simulink model "T3_updatesolarpart"  (R2022b)
settings: Solver=VariableStepAuto  StartTime=0.0  StopTime=10.0  RelTol=1e-3
undefined symbols (not defined in the file): High, Low
libraries: fl_lib x101, nesl_utility x52, simulink x14, ee_lib x5, slpidlib x2, eePwmGenerator x1
(part 2 of 3)

== system T3_updatesolarpart/Household 9 ==
  Current Sensor : fl_lib/Electrical/Electrical Sensors/Current Sensor
  PS-Simulink Converter : nesl_utility/PS-Simulink Converter  PhysicalDomain=network_engine_domain  SubClassName=ps_output  LeftPortType=input  RightPortType=output  PseudoPeriodic=off  Frequencies=[]  VectorFormat=inherit  Unit=inherit  AffineConversion=off
  PS-Simulink Converter1 : nesl_utility/PS-Simulink Converter  PhysicalDomain=network_engine_domain  SubClassName=ps_output  LeftPortType=input  RightPortType=output  PseudoPeriodic=off  Frequencies=[]  VectorFormat=inherit  Unit=inherit  AffineConversion=off
  Product : Product
  "Residential power " : simulink/Sources/Repeating Sequence Interpolated  OutValues=[2.8 2.5 2 2 2.2 2.5 2.8 3.4 3.6 3.8 4 4 4 4 4 4 4 4 4 4 3.8 3.5 3.2 3]*1000  TimeValues=[0 1 2 3 4 5 6 7 8 9 10 11 12 13 14 15 16 17 18 19 20 21 22 23]  LookUpMeth=Interpolation-Use End Values  tsamp=1e-4  OutMin=[]  OutMax=[]  OutDataTypeStr=double  OutputDataTypeScalingMode=double  OutDataType=fixdt(0,8)  OutScaling=2^-10
  Simscape Component : SimscapeComponentBlock  SourceFile=ResidentialPowerLoad  ComponentPath=ResidentialPowerLoad  ComponentVariants="[\"ResidentialPowerLoad\"]"  ComponentVariantNames="[\"ResidentialPowerLoad\"]"  ClassName=ResidentialPowerLoad  SchemaVersion=1  i_specify=off  i_priority=None  i=0 A  i_nominal_specify=off  i_nominal_unit=A  i_nominal_value=1  v_specify=off  v_priority=None  v=0 V  v_nominal_specify=off  v_nominal_unit=V  v_nominal_value=1
      settings: CopyFcn=simscape.engine.sli.internal.componentblockcallback(gcbh,'COPY')  PreCopyFcn=simscape.engine.sli.internal.componentblockcallback(gcbh,'PRECOPY')  PreDeleteFcn=simscape.engine.sli.internal.componentblockcallback(gcbh,'PREDELETE')  InternalSimscapePortConfiguration="{\"Bottom\":[],\"Left\":[{\"id\":\"Power\",\"label\":\"P\",\"type\":\"input\"},{\"id\":\"p\",\"label\":\"+\",\"type\":\"foundation.electrical.electrical\"}],\"Right\":[{\"id\":\"n\",\"label\":\"-\",\"type\":\"foundation.electrical.electrical\"}],\"Top\":[]}"
      mask Type: ResidentialPowerLoad
      mask Display: color('red');plot([0 1 1 0 0],[0 0 1 1 0]);plot([0.7,1],[1,0.7]);plot(-2,-1.75);plot(3, 1);disp('\n.ssc\nUnresolved')
  Simscape Bus1 : SimscapeBus  HierarchyStrings=High;Low
  Simulink-PS Converter : nesl_utility/Simulink-PS Converter  PhysicalDomain=network_engine_domain  SubClassName=ps_input  LeftPortType=input  RightPortType=output  PseudoPeriodic=off  Frequencies=[]  NoiseDistribution=none  NoiseParameters=[]  Unit=1  AffineConversion=off  FilteringAndDerivatives=provide  SimscapeFilterOrder=1  InputFilterTimeConstant=0.001  UdotUserProvided=0
  Terminator : Terminator
  Voltage Sensor : fl_lib/Electrical/Electrical Sensors/Voltage Sensor
  ResidentialOut : PMIOPort  Side=Right
  wires:
  Product/1 -> Terminator/1  "power"
  PS-Simulink Converter1/1 -> Product/1  "current"
  PS-Simulink Converter/1 -> Product/2  "voltage"
  "Residential power "/1 -> Simulink-PS Converter/1
  connections:
  Current Sensor/RConn1 -- PS-Simulink Converter1/LConn1
  Current Sensor/LConn1 -- Simscape Bus1/LConn1
  Simulink-PS Converter/RConn1 -- Simscape Component/LConn1
  Voltage Sensor/RConn1 -- PS-Simulink Converter/LConn1
  Voltage Sensor/LConn1 -- Current Sensor/RConn2 -- Simscape Component/LConn2
  ResidentialOut/RConn1 -- Simscape Bus1/RConn1
  Simscape Component/RConn1 -- Simscape Bus1/LConn2 -- Voltage Sensor/RConn2

== system T3_updatesolarpart/Line1 ==
  Resistor : fl_lib/Electrical/Electrical Elements/Resistor  R=rho*l/A Ohm  i_specify=off  i_priority=None  i=0 A  i_nominal_specify=off  i_nominal_unit=A  i_nominal_value=1  v_specify=off  v_priority=None  v=0 V  v_nominal_specify=off  v_nominal_unit=V  v_nominal_value=1
  Resistor1 : fl_lib/Electrical/Electrical Elements/Resistor  R=rho*l/A Ohm  i_specify=off  i_priority=None  i=0 A  i_nominal_specify=off  i_nominal_unit=A  i_nominal_value=1  v_specify=off  v_priority=None  v=0 V  v_nominal_specify=off  v_nominal_unit=V  v_nominal_value=1
  Simscape Bus2 : SimscapeBus  HierarchyStrings=High;Low
  Simscape Bus3 : SimscapeBus  HierarchyStrings=High;Low
  In : PMIOPort  Side=Left
  Out : PMIOPort  Port=2  Side=Right
  connections:
  Simscape Bus2/LConn1 -- Resistor/LConn1
  Simscape Bus3/LConn2 -- Resistor1/RConn1
  Simscape Bus2/RConn1 -- In/RConn1
  Simscape Bus3/LConn1 -- Resistor/RConn1
  Resistor1/LConn1 -- Simscape Bus2/LConn2
  Simscape Bus3/RConn1 -- Out/RConn1

== system T3_updatesolarpart/Line10 ==
  Resistor : fl_lib/Electrical/Electrical Elements/Resistor  R=rho*l/A Ohm  i_specify=off  i_priority=None  i=0 A  i_nominal_specify=off  i_nominal_unit=A  i_nominal_value=1  v_specify=off  v_priority=None  v=0 V  v_nominal_specify=off  v_nominal_unit=V  v_nominal_value=1
  Resistor1 : fl_lib/Electrical/Electrical Elements/Resistor  R=rho*l/A Ohm  i_specify=off  i_priority=None  i=0 A  i_nominal_specify=off  i_nominal_unit=A  i_nominal_value=1  v_specify=off  v_priority=None  v=0 V  v_nominal_specify=off  v_nominal_unit=V  v_nominal_value=1
  Simscape Bus2 : SimscapeBus  HierarchyStrings=High;Low
  Simscape Bus3 : SimscapeBus  HierarchyStrings=High;Low
  In : PMIOPort  Side=Left
  Out : PMIOPort  Port=2  Side=Right
  connections:
  Simscape Bus2/LConn1 -- Resistor/LConn1
  Simscape Bus3/LConn2 -- Resistor1/RConn1
  Simscape Bus2/RConn1 -- In/RConn1
  Simscape Bus3/LConn1 -- Resistor/RConn1
  Resistor1/LConn1 -- Simscape Bus2/LConn2
  Simscape Bus3/RConn1 -- Out/RConn1

== system T3_updatesolarpart/Line11 ==
  Resistor : fl_lib/Electrical/Electrical Elements/Resistor  R=rho*l/A Ohm  i_specify=off  i_priority=None  i=0 A  i_nominal_specify=off  i_nominal_unit=A  i_nominal_value=1  v_specify=off  v_priority=None  v=0 V  v_nominal_specify=off  v_nominal_unit=V  v_nominal_value=1
  Resistor1 : fl_lib/Electrical/Electrical Elements/Resistor  R=rho*l/A Ohm  i_specify=off  i_priority=None  i=0 A  i_nominal_specify=off  i_nominal_unit=A  i_nominal_value=1  v_specify=off  v_priority=None  v=0 V  v_nominal_specify=off  v_nominal_unit=V  v_nominal_value=1
  Simscape Bus2 : SimscapeBus  HierarchyStrings=High;Low
  Simscape Bus3 : SimscapeBus  HierarchyStrings=High;Low
  In : PMIOPort  Side=Left
  Out : PMIOPort  Port=2  Side=Right
  connections:
  Simscape Bus3/RConn1 -- Out/RConn1
  Resistor1/LConn1 -- Simscape Bus2/LConn2
  Simscape Bus3/LConn1 -- Resistor/RConn1
  Simscape Bus2/RConn1 -- In/RConn1
  Simscape Bus3/LConn2 -- Resistor1/RConn1
  Simscape Bus2/LConn1 -- Resistor/LConn1

== system T3_updatesolarpart/Line12 ==
  Resistor : fl_lib/Electrical/Electrical Elements/Resistor  R=rho*l/A Ohm  i_specify=off  i_priority=None  i=0 A  i_nominal_specify=off  i_nominal_unit=A  i_nominal_value=1  v_specify=off  v_priority=None  v=0 V  v_nominal_specify=off  v_nominal_unit=V  v_nominal_value=1
  Resistor1 : fl_lib/Electrical/Electrical Elements/Resistor  R=rho*l/A Ohm  i_specify=off  i_priority=None  i=0 A  i_nominal_specify=off  i_nominal_unit=A  i_nominal_value=1  v_specify=off  v_priority=None  v=0 V  v_nominal_specify=off  v_nominal_unit=V  v_nominal_value=1
  Simscape Bus2 : SimscapeBus  HierarchyStrings=High;Low
  Simscape Bus3 : SimscapeBus  HierarchyStrings=High;Low
  In : PMIOPort  Side=Left
  Out : PMIOPort  Port=2  Side=Right
  connections:
  Simscape Bus3/RConn1 -- Out/RConn1
  Resistor1/LConn1 -- Simscape Bus2/LConn2
  Simscape Bus3/LConn1 -- Resistor/RConn1
  Simscape Bus2/RConn1 -- In/RConn1
  Simscape Bus3/LConn2 -- Resistor1/RConn1
  Simscape Bus2/LConn1 -- Resistor/LConn1

== system T3_updatesolarpart/Line13 ==
  Resistor : fl_lib/Electrical/Electrical Elements/Resistor  R=rho*l/A Ohm  i_specify=off  i_priority=None  i=0 A  i_nominal_specify=off  i_nominal_unit=A  i_nominal_value=1  v_specify=off  v_priority=None  v=0 V  v_nominal_specify=off  v_nominal_unit=V  v_nominal_value=1
  Resistor1 : fl_lib/Electrical/Electrical Elements/Resistor  R=rho*l/A Ohm  i_specify=off  i_priority=None  i=0 A  i_nominal_specify=off  i_nominal_unit=A  i_nominal_value=1  v_specify=off  v_priority=None  v=0 V  v_nominal_specify=off  v_nominal_unit=V  v_nominal_value=1
  Simscape Bus2 : SimscapeBus  HierarchyStrings=High;Low
  Simscape Bus3 : SimscapeBus  HierarchyStrings=High;Low
  In : PMIOPort  Side=Left
  Out : PMIOPort  Port=2  Side=Right
  connections:
  Simscape Bus2/LConn1 -- Resistor/LConn1
  Simscape Bus3/LConn2 -- Resistor1/RConn1
  Simscape Bus2/RConn1 -- In/RConn1
  Simscape Bus3/LConn1 -- Resistor/RConn1
  Resistor1/LConn1 -- Simscape Bus2/LConn2
  Simscape Bus3/RConn1 -- Out/RConn1

== system T3_updatesolarpart/Line14 ==
  Resistor : fl_lib/Electrical/Electrical Elements/Resistor  R=rho*l/A Ohm  i_specify=off  i_priority=None  i=0 A  i_nominal_specify=off  i_nominal_unit=A  i_nominal_value=1  v_specify=off  v_priority=None  v=0 V  v_nominal_specify=off  v_nominal_unit=V  v_nominal_value=1
  Resistor1 : fl_lib/Electrical/Electrical Elements/Resistor  R=rho*l/A Ohm  i_specify=off  i_priority=None  i=0 A  i_nominal_specify=off  i_nominal_unit=A  i_nominal_value=1  v_specify=off  v_priority=None  v=0 V  v_nominal_specify=off  v_nominal_unit=V  v_nominal_value=1
  Simscape Bus2 : SimscapeBus  HierarchyStrings=High;Low
  Simscape Bus3 : SimscapeBus  HierarchyStrings=High;Low
  In : PMIOPort  Side=Left
  Out : PMIOPort  Port=2  Side=Right
  connections:
  Simscape Bus3/RConn1 -- Out/RConn1
  Resistor1/LConn1 -- Simscape Bus2/LConn2
  Simscape Bus3/LConn1 -- Resistor/RConn1
  Simscape Bus2/RConn1 -- In/RConn1
  Simscape Bus3/LConn2 -- Resistor1/RConn1
  Simscape Bus2/LConn1 -- Resistor/LConn1

== system T3_updatesolarpart/Line15 ==
  Resistor : fl_lib/Electrical/Electrical Elements/Resistor  R=rho*l/A Ohm  i_specify=off  i_priority=None  i=0 A  i_nominal_specify=off  i_nominal_unit=A  i_nominal_value=1  v_specify=off  v_priority=None  v=0 V  v_nominal_specify=off  v_nominal_unit=V  v_nominal_value=1
  Resistor1 : fl_lib/Electrical/Electrical Elements/Resistor  R=rho*l/A Ohm  i_specify=off  i_priority=None  i=0 A  i_nominal_specify=off  i_nominal_unit=A  i_nominal_value=1  v_specify=off  v_priority=None  v=0 V  v_nominal_specify=off  v_nominal_unit=V  v_nominal_value=1
  Simscape Bus2 : SimscapeBus  HierarchyStrings=High;Low
  Simscape Bus3 : SimscapeBus  HierarchyStrings=High;Low
  In : PMIOPort  Side=Left
  Out : PMIOPort  Port=2  Side=Right
  connections:
  Simscape Bus2/LConn1 -- Resistor/LConn1
  Simscape Bus3/LConn2 -- Resistor1/RConn1
  Simscape Bus2/RConn1 -- In/RConn1
  Simscape Bus3/LConn1 -- Resistor/RConn1
  Resistor1/LConn1 -- Simscape Bus2/LConn2
  Simscape Bus3/RConn1 -- Out/RConn1

== system T3_updatesolarpart/Line16 ==
  Resistor : fl_lib/Electrical/Electrical Elements/Resistor  R=rho*l/A Ohm  i_specify=off  i_priority=None  i=0 A  i_nominal_specify=off  i_nominal_unit=A  i_nominal_value=1  v_specify=off  v_priority=None  v=0 V  v_nominal_specify=off  v_nominal_unit=V  v_nominal_value=1
  Resistor1 : fl_lib/Electrical/Electrical Elements/Resistor  R=rho*l/A Ohm  i_specify=off  i_priority=None  i=0 A  i_nominal_specify=off  i_nominal_unit=A  i_nominal_value=1  v_specify=off  v_priority=None  v=0 V  v_nominal_specify=off  v_nominal_unit=V  v_nominal_value=1
  Simscape Bus2 : SimscapeBus  HierarchyStrings=High;Low
  Simscape Bus3 : SimscapeBus  HierarchyStrings=High;Low
  In : PMIOPort  Side=Left
  Out : PMIOPort  Port=2  Side=Right
  connections:
  Simscape Bus2/LConn1 -- Resistor/LConn1
  Simscape Bus3/LConn2 -- Resistor1/RConn1
  Simscape Bus2/RConn1 -- In/RConn1
  Simscape Bus3/LConn1 -- Resistor/RConn1
  Resistor1/LConn1 -- Simscape Bus2/LConn2
  Simscape Bus3/RConn1 -- Out/RConn1

== system T3_updatesolarpart/Line17 ==
  Resistor : fl_lib/Electrical/Electrical Elements/Resistor  R=rho*l/A Ohm  i_specify=off  i_priority=None  i=0 A  i_nominal_specify=off  i_nominal_unit=A  i_nominal_value=1  v_specify=off  v_priority=None  v=0 V  v_nominal_specify=off  v_nominal_unit=V  v_nominal_value=1
  Resistor1 : fl_lib/Electrical/Electrical Elements/Resistor  R=rho*l/A Ohm  i_specify=off  i_priority=None  i=0 A  i_nominal_specify=off  i_nominal_unit=A  i_nominal_value=1  v_specify=off  v_priority=None  v=0 V  v_nominal_specify=off  v_nominal_unit=V  v_nominal_value=1
  Simscape Bus2 : SimscapeBus  HierarchyStrings=High;Low
  Simscape Bus3 : SimscapeBus  HierarchyStrings=High;Low
  In : PMIOPort  Side=Left
  Out : PMIOPort  Port=2  Side=Right
  connections:
  Simscape Bus3/RConn1 -- Out/RConn1
  Resistor1/LConn1 -- Simscape Bus2/LConn2
  Simscape Bus3/LConn1 -- Resistor/RConn1
  Simscape Bus2/RConn1 -- In/RConn1
  Simscape Bus3/LConn2 -- Resistor1/RConn1
  Simscape Bus2/LConn1 -- Resistor/LConn1

== system T3_updatesolarpart/Line18 ==
  Resistor : fl_lib/Electrical/Electrical Elements/Resistor  R=rho*l/A Ohm  i_specify=off  i_priority=None  i=0 A  i_nominal_specify=off  i_nominal_unit=A  i_nominal_value=1  v_specify=off  v_priority=None  v=0 V  v_nominal_specify=off  v_nominal_unit=V  v_nominal_value=1
  Resistor1 : fl_lib/Electrical/Electrical Elements/Resistor  R=rho*l/A Ohm  i_specify=off  i_priority=None  i=0 A  i_nominal_specify=off  i_nominal_unit=A  i_nominal_value=1  v_specify=off  v_priority=None  v=0 V  v_nominal_specify=off  v_nominal_unit=V  v_nominal_value=1
  Simscape Bus2 : SimscapeBus  HierarchyStrings=High;Low
  Simscape Bus3 : SimscapeBus  HierarchyStrings=High;Low
  In : PMIOPort  Side=Left
  Out : PMIOPort  Port=2  Side=Right
  connections:
  Simscape Bus3/RConn1 -- Out/RConn1
  Resistor1/LConn1 -- Simscape Bus2/LConn2
  Simscape Bus3/LConn1 -- Resistor/RConn1
  Simscape Bus2/RConn1 -- In/RConn1
  Simscape Bus3/LConn2 -- Resistor1/RConn1
  Simscape Bus2/LConn1 -- Resistor/LConn1

== system T3_updatesolarpart/Line19 ==
  Resistor : fl_lib/Electrical/Electrical Elements/Resistor  R=rho*l/A Ohm  i_specify=off  i_priority=None  i=0 A  i_nominal_specify=off  i_nominal_unit=A  i_nominal_value=1  v_specify=off  v_priority=None  v=0 V  v_nominal_specify=off  v_nominal_unit=V  v_nominal_value=1
  Resistor1 : fl_lib/Electrical/Electrical Elements/Resistor  R=rho*l/A Ohm  i_specify=off  i_priority=None  i=0 A  i_nominal_specify=off  i_nominal_unit=A  i_nominal_value=1  v_specify=off  v_priority=None  v=0 V  v_nominal_specify=off  v_nominal_unit=V  v_nominal_value=1
  Simscape Bus2 : SimscapeBus  HierarchyStrings=High;Low
  Simscape Bus3 : SimscapeBus  HierarchyStrings=High;Low
  In : PMIOPort  Side=Left
  Out : PMIOPort  Port=2  Side=Right
  connections:
  Simscape Bus2/LConn1 -- Resistor/LConn1
  Simscape Bus3/LConn2 -- Resistor1/RConn1
  Simscape Bus2/RConn1 -- In/RConn1
  Simscape Bus3/LConn1 -- Resistor/RConn1
  Resistor1/LConn1 -- Simscape Bus2/LConn2
  Simscape Bus3/RConn1 -- Out/RConn1

== system T3_updatesolarpart/Line2 ==
  Resistor : fl_lib/Electrical/Electrical Elements/Resistor  R=rho*l/A Ohm  i_specify=off  i_priority=None  i=0 A  i_nominal_specify=off  i_nominal_unit=A  i_nominal_value=1  v_specify=off  v_priority=None  v=0 V  v_nominal_specify=off  v_nominal_unit=V  v_nominal_value=1
  Resistor1 : fl_lib/Electrical/Electrical Elements/Resistor  R=rho*l/A Ohm  i_specify=off  i_priority=None  i=0 A  i_nominal_specify=off  i_nominal_unit=A  i_nominal_value=1  v_specify=off  v_priority=None  v=0 V  v_nominal_specify=off  v_nominal_unit=V  v_nominal_value=1
  Simscape Bus2 : SimscapeBus  HierarchyStrings=High;Low
  Simscape Bus3 : SimscapeBus  HierarchyStrings=High;Low
  In : PMIOPort  Side=Left
  Out : PMIOPort  Port=2  Side=Right
  connections:
  Simscape Bus3/RConn1 -- Out/RConn1
  Resistor1/LConn1 -- Simscape Bus2/LConn2
  Simscape Bus3/LConn1 -- Resistor/RConn1
  Simscape Bus2/RConn1 -- In/RConn1
  Simscape Bus3/LConn2 -- Resistor1/RConn1
  Simscape Bus2/LConn1 -- Resistor/LConn1

== system T3_updatesolarpart/Line20 ==
  Resistor : fl_lib/Electrical/Electrical Elements/Resistor  R=rho*l/A Ohm  i_specify=off  i_priority=None  i=0 A  i_nominal_specify=off  i_nominal_unit=A  i_nominal_value=1  v_specify=off  v_priority=None  v=0 V  v_nominal_specify=off  v_nominal_unit=V  v_nominal_value=1
  Resistor1 : fl_lib/Electrical/Electrical Elements/Resistor  R=rho*l/A Ohm  i_specify=off  i_priority=None  i=0 A  i_nominal_specify=off  i_nominal_unit=A  i_nominal_value=1  v_specify=off  v_priority=None  v=0 V  v_nominal_specify=off  v_nominal_unit=V  v_nominal_value=1
  Simscape Bus2 : SimscapeBus  HierarchyStrings=High;Low
  Simscape Bus3 : SimscapeBus  HierarchyStrings=High;Low
  In : PMIOPort  Side=Left
  Out : PMIOPort  Port=2  Side=Right
  connections:
  Simscape Bus3/RConn1 -- Out/RConn1
  Resistor1/LConn1 -- Simscape Bus2/LConn2
  Simscape Bus3/LConn1 -- Resistor/RConn1
  Simscape Bus2/RConn1 -- In/RConn1
  Simscape Bus3/LConn2 -- Resistor1/RConn1
  Simscape Bus2/LConn1 -- Resistor/LConn1

== system T3_updatesolarpart/Line3 ==
  Resistor : fl_lib/Electrical/Electrical Elements/Resistor  R=rho*l/A Ohm  i_specify=off  i_priority=None  i=0 A  i_nominal_specify=off  i_nominal_unit=A  i_nominal_value=1  v_specify=off  v_priority=None  v=0 V  v_nominal_specify=off  v_nominal_unit=V  v_nominal_value=1
  Resistor1 : fl_lib/Electrical/Electrical Elements/Resistor  R=rho*l/A Ohm  i_specify=off  i_priority=None  i=0 A  i_nominal_specify=off  i_nominal_unit=A  i_nominal_value=1  v_specify=off  v_priority=None  v=0 V  v_nominal_specify=off  v_nominal_unit=V  v_nominal_value=1
  Simscape Bus2 : SimscapeBus  HierarchyStrings=High;Low
  Simscape Bus3 : SimscapeBus  HierarchyStrings=High;Low
  In : PMIOPort  Side=Left
  Out : PMIOPort  Port=2  Side=Right
  connections:
  Simscape Bus2/LConn1 -- Resistor/LConn1
  Simscape Bus3/LConn2 -- Resistor1/RConn1
  Simscape Bus2/RConn1 -- In/RConn1
  Simscape Bus3/LConn1 -- Resistor/RConn1
  Resistor1/LConn1 -- Simscape Bus2/LConn2
  Simscape Bus3/RConn1 -- Out/RConn1

== system T3_updatesolarpart/Line4 ==
  Resistor : fl_lib/Electrical/Electrical Elements/Resistor  R=rho*l/A Ohm  i_specify=off  i_priority=None  i=0 A  i_nominal_specify=off  i_nominal_unit=A  i_nominal_value=1  v_specify=off  v_priority=None  v=0 V  v_nominal_specify=off  v_nominal_unit=V  v_nominal_value=1
  Resistor1 : fl_lib/Electrical/Electrical Elements/Resistor  R=rho*l/A Ohm  i_specify=off  i_priority=None  i=0 A  i_nominal_specify=off  i_nominal_unit=A  i_nominal_value=1  v_specify=off  v_priority=None  v=0 V  v_nominal_specify=off  v_nominal_unit=V  v_nominal_value=1
  Simscape Bus2 : SimscapeBus  HierarchyStrings=High;Low
  Simscape Bus3 : SimscapeBus  HierarchyStrings=High;Low
  In : PMIOPort  Side=Left
  Out : PMIOPort  Port=2  Side=Right
  connections:
  Simscape Bus3/RConn1 -- Out/RConn1
  Resistor1/LConn1 -- Simscape Bus2/LConn2
  Simscape Bus3/LConn1 -- Resistor/RConn1
  Simscape Bus2/RConn1 -- In/RConn1
  Simscape Bus3/LConn2 -- Resistor1/RConn1
  Simscape Bus2/LConn1 -- Resistor/LConn1

== system T3_updatesolarpart/Line5 ==
  Resistor : fl_lib/Electrical/Electrical Elements/Resistor  R=rho*l/A Ohm  i_specify=off  i_priority=None  i=0 A  i_nominal_specify=off  i_nominal_unit=A  i_nominal_value=1  v_specify=off  v_priority=None  v=0 V  v_nominal_specify=off  v_nominal_unit=V  v_nominal_value=1
  Resistor1 : fl_lib/Electrical/Electrical Elements/Resistor  R=rho*l/A Ohm  i_specify=off  i_priority=None  i=0 A  i_nominal_specify=off  i_nominal_unit=A  i_nominal_value=1  v_specify=off  v_priority=None  v=0 V  v_nominal_specify=off  v_nominal_unit=V  v_nominal_value=1
  Simscape Bus2 : SimscapeBus  HierarchyStrings=High;Low
  Simscape Bus3 : SimscapeBus  HierarchyStrings=High;Low
  In : PMIOPort  Side=Left
  Out : PMIOPort  Port=2  Side=Right
  connections:
  Simscape Bus2/LConn1 -- Resistor/LConn1
  Simscape Bus3/LConn2 -- Resistor1/RConn1
  Simscape Bus2/RConn1 -- In/RConn1
  Simscape Bus3/LConn1 -- Resistor/RConn1
  Resistor1/LConn1 -- Simscape Bus2/LConn2
  Simscape Bus3/RConn1 -- Out/RConn1

== system T3_updatesolarpart/Line6 ==
  Resistor : fl_lib/Electrical/Electrical Elements/Resistor  R=rho*l/A Ohm  i_specify=off  i_priority=None  i=0 A  i_nominal_specify=off  i_nominal_unit=A  i_nominal_value=1  v_specify=off  v_priority=None  v=0 V  v_nominal_specify=off  v_nominal_unit=V  v_nominal_value=1
  Resistor1 : fl_lib/Electrical/Electrical Elements/Resistor  R=rho*l/A Ohm  i_specify=off  i_priority=None  i=0 A  i_nominal_specify=off  i_nominal_unit=A  i_nominal_value=1  v_specify=off  v_priority=None  v=0 V  v_nominal_specify=off  v_nominal_unit=V  v_nominal_value=1
  Simscape Bus2 : SimscapeBus  HierarchyStrings=High;Low
  Simscape Bus3 : SimscapeBus  HierarchyStrings=High;Low
  In : PMIOPort  Side=Left
  Out : PMIOPort  Port=2  Side=Right
  connections:
  Simscape Bus3/RConn1 -- Out/RConn1
  Resistor1/LConn1 -- Simscape Bus2/LConn2
  Simscape Bus3/LConn1 -- Resistor/RConn1
  Simscape Bus2/RConn1 -- In/RConn1
  Simscape Bus3/LConn2 -- Resistor1/RConn1
  Simscape Bus2/LConn1 -- Resistor/LConn1

== system T3_updatesolarpart/Line7 ==
  Resistor : fl_lib/Electrical/Electrical Elements/Resistor  R=rho*l/A Ohm  i_specify=off  i_priority=None  i=0 A  i_nominal_specify=off  i_nominal_unit=A  i_nominal_value=1  v_specify=off  v_priority=None  v=0 V  v_nominal_specify=off  v_nominal_unit=V  v_nominal_value=1
  Resistor1 : fl_lib/Electrical/Electrical Elements/Resistor  R=rho*l/A Ohm  i_specify=off  i_priority=None  i=0 A  i_nominal_specify=off  i_nominal_unit=A  i_nominal_value=1  v_specify=off  v_priority=None  v=0 V  v_nominal_specify=off  v_nominal_unit=V  v_nominal_value=1
  Simscape Bus2 : SimscapeBus  HierarchyStrings=High;Low
  Simscape Bus3 : SimscapeBus  HierarchyStrings=High;Low
  In : PMIOPort  Side=Left
  Out : PMIOPort  Port=2  Side=Right
  connections:
  Simscape Bus2/LConn1 -- Resistor/LConn1
  Simscape Bus3/LConn2 -- Resistor1/RConn1
  Simscape Bus2/RConn1 -- In/RConn1
  Simscape Bus3/LConn1 -- Resistor/RConn1
  Resistor1/LConn1 -- Simscape Bus2/LConn2
  Simscape Bus3/RConn1 -- Out/RConn1

== system T3_updatesolarpart/Line8 ==
  Resistor : fl_lib/Electrical/Electrical Elements/Resistor  R=rho*l/A Ohm  i_specify=off  i_priority=None  i=0 A  i_nominal_specify=off  i_nominal_unit=A  i_nominal_value=1  v_specify=off  v_priority=None  v=0 V  v_nominal_specify=off  v_nominal_unit=V  v_nominal_value=1
  Resistor1 : fl_lib/Electrical/Electrical Elements/Resistor  R=rho*l/A Ohm  i_specify=off  i_priority=None  i=0 A  i_nominal_specify=off  i_nominal_unit=A  i_nominal_value=1  v_specify=off  v_priority=None  v=0 V  v_nominal_specify=off  v_nominal_unit=V  v_nominal_value=1
  Simscape Bus2 : SimscapeBus  HierarchyStrings=High;Low
  Simscape Bus3 : SimscapeBus  HierarchyStrings=High;Low
  In : PMIOPort  Side=Left
  Out : PMIOPort  Port=2  Side=Right
  connections:
  Simscape Bus2/LConn1 -- Resistor/LConn1
  Simscape Bus3/LConn2 -- Resistor1/RConn1
  Simscape Bus2/RConn1 -- In/RConn1
  Simscape Bus3/LConn1 -- Resistor/RConn1
  Resistor1/LConn1 -- Simscape Bus2/LConn2
  Simscape Bus3/RConn1 -- Out/RConn1

== system T3_updatesolarpart/Line9 ==
  Resistor : fl_lib/Electrical/Electrical Elements/Resistor  R=rho*l/A Ohm  i_specify=off  i_priority=None  i=0 A  i_nominal_specify=off  i_nominal_unit=A  i_nominal_value=1  v_specify=off  v_priority=None  v=0 V  v_nominal_specify=off  v_nominal_unit=V  v_nominal_value=1
  Resistor1 : fl_lib/Electrical/Electrical Elements/Resistor  R=rho*l/A Ohm  i_specify=off  i_priority=None  i=0 A  i_nominal_specify=off  i_nominal_unit=A  i_nominal_value=1  v_specify=off  v_priority=None  v=0 V  v_nominal_specify=off  v_nominal_unit=V  v_nominal_value=1
  Simscape Bus2 : SimscapeBus  HierarchyStrings=High;Low
  Simscape Bus3 : SimscapeBus  HierarchyStrings=High;Low
  In : PMIOPort  Side=Left
  Out : PMIOPort  Port=2  Side=Right
  connections:
  Simscape Bus3/RConn1 -- Out/RConn1
  Resistor1/LConn1 -- Simscape Bus2/LConn2
  Simscape Bus3/LConn1 -- Resistor/RConn1
  Simscape Bus2/RConn1 -- In/RConn1
  Simscape Bus3/LConn2 -- Resistor1/RConn1
  Simscape Bus2/LConn1 -- Resistor/LConn1

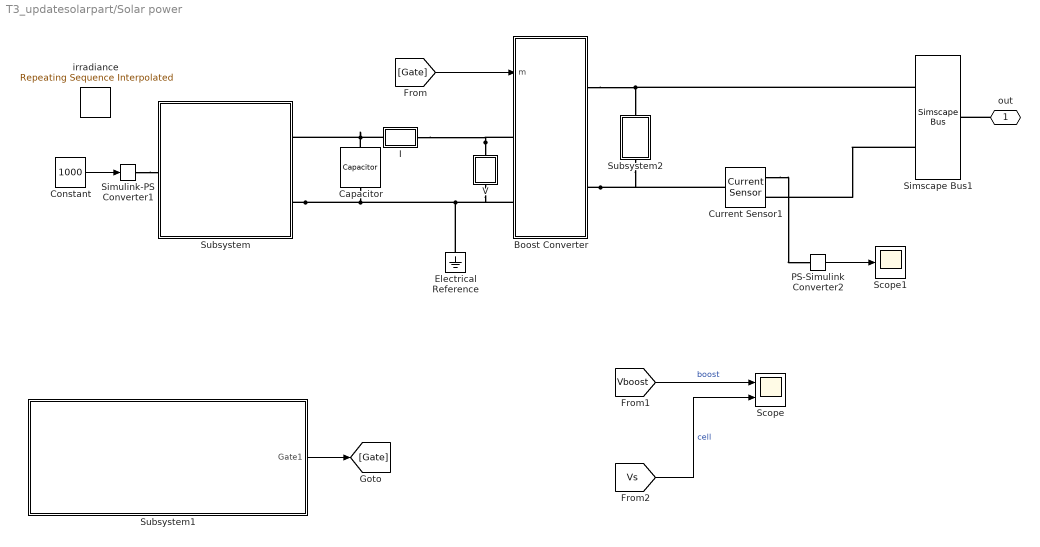
== system T3_updatesolarpart/Solar power ==
  Boost Converter : Subsystem  VariantControl=boostCircuit == 1
  Capacitor : fl_lib/Electrical/Electrical Elements/Capacitor  c=1e-3 F  r=1e-6 Ohm  g=0 1/Ohm  i_specify=off  i_priority=None  i=0 A  i_nominal_specify=off  i_nominal_unit=A  i_nominal_value=1  v_specify=off  v_priority=None  v=0 V  v_nominal_specify=off  v_nominal_unit=V  v_nominal_value=1  vc_specify=off  vc_priority=High  vc=0 V  vc_nominal_specify=off  vc_nominal_unit=V  vc_nominal_value=1
  Constant : Constant  Value=1000  SampleTime=20e3
  Current Sensor1 : fl_lib/Electrical/Electrical Sensors/Current Sensor
  Electrical Reference : fl_lib/Electrical/Electrical Elements/Electrical Reference
  I : Subsystem
  PS-Simulink Converter2 : nesl_utility/PS-Simulink Converter  PhysicalDomain=network_engine_domain  SubClassName=ps_output  LeftPortType=input  RightPortType=output  PseudoPeriodic=off  Frequencies=[]  VectorFormat=inherit  Unit=inherit  AffineConversion=off
  Scope : Scope  NumInputPorts=2
  Scope1 : Scope
  Simscape Bus1 : SimscapeBus  HierarchyStrings=High;Low
  Simulink-PS Converter1 : nesl_utility/Simulink-PS Converter  PhysicalDomain=network_engine_domain  SubClassName=ps_input  LeftPortType=input  RightPortType=output  PseudoPeriodic=off  Frequencies=[]  NoiseDistribution=none  NoiseParameters=[]  Unit=1  AffineConversion=off  FilteringAndDerivatives=provide  SimscapeFilterOrder=1  InputFilterTimeConstant=0.001  UdotUserProvided=0
  Subsystem : Subsystem
  Subsystem1 : Subsystem
  Subsystem2 : Subsystem
  V : Subsystem
  "irradiance " : simulink/Sources/Repeating Sequence Interpolated  OutValues=[0 0 1 1 2 2 3 3 4 4 5 5 6 6 5 5 4 4 3 3 2 2 1 1]*200  TimeValues=[0 1 2 3 4 5 6 7 8 9 10 11 12 13 14 15 16 17 18 19 20 21 22 23]  LookUpMeth=Interpolation-Use End Values  tsamp=1e-4  OutMin=[]  OutMax=[]  OutDataTypeStr=double  OutputDataTypeScalingMode=double  OutDataType=fixdt(0,8)  OutScaling=2^-10
  out : PMIOPort  Side=Left
  wires:
  [Vs] -> Scope/2  "cell"
  [Gate] -> Boost Converter/1(m)
  [Vboost] -> Scope/1  "boost"
  Constant/1 -> Simulink-PS Converter1/1
  Subsystem1/1(Gate1) -> [Gate]
  PS-Simulink Converter2/1 -> Scope1/1
  connections:
  out/RConn1 -- Simscape Bus1/RConn1
  Subsystem/RConn2 -- Capacitor/RConn1 -- Electrical Reference/LConn1 -- V/RConn1 -- Boost Converter/LConn2
  Boost Converter/RConn2 -- Subsystem2/RConn1 -- Current Sensor1/LConn1
  V/LConn1 -- I/RConn1 -- Boost Converter/LConn1
  I/LConn1 -- Capacitor/LConn1 -- Subsystem/RConn1
  Boost Converter/RConn1 -- Simscape Bus1/LConn1 -- Subsystem2/LConn1
  Simulink-PS Converter1/RConn1 -- Subsystem/LConn1
  Current Sensor1/RConn1 -- PS-Simulink Converter2/LConn1
  Simscape Bus1/LConn2 -- Current Sensor1/RConn2

== system T3_updatesolarpart/Subsystem10 ==
  Resistor : fl_lib/Electrical/Electrical Elements/Resistor  R=rho*l/A Ohm  i_specify=off  i_priority=None  i=0 A  i_nominal_specify=off  i_nominal_unit=A  i_nominal_value=1  v_specify=off  v_priority=None  v=0 V  v_nominal_specify=off  v_nominal_unit=V  v_nominal_value=1
  Resistor1 : fl_lib/Electrical/Electrical Elements/Resistor  R=rho*l/A Ohm  i_specify=off  i_priority=None  i=0 A  i_nominal_specify=off  i_nominal_unit=A  i_nominal_value=1  v_specify=off  v_priority=None  v=0 V  v_nominal_specify=off  v_nominal_unit=V  v_nominal_value=1
  Simscape Bus2 : SimscapeBus  HierarchyStrings=High;Low
  Simscape Bus3 : SimscapeBus  HierarchyStrings=High;Low
  In : PMIOPort  Side=Left
  Out : PMIOPort  Port=2  Side=Right
  connections:
  Simscape Bus3/RConn1 -- Out/RConn1
  Resistor1/LConn1 -- Simscape Bus2/LConn2
  Simscape Bus3/LConn1 -- Resistor/RConn1
  Simscape Bus2/RConn1 -- In/RConn1
  Simscape Bus3/LConn2 -- Resistor1/RConn1
  Simscape Bus2/LConn1 -- Resistor/LConn1

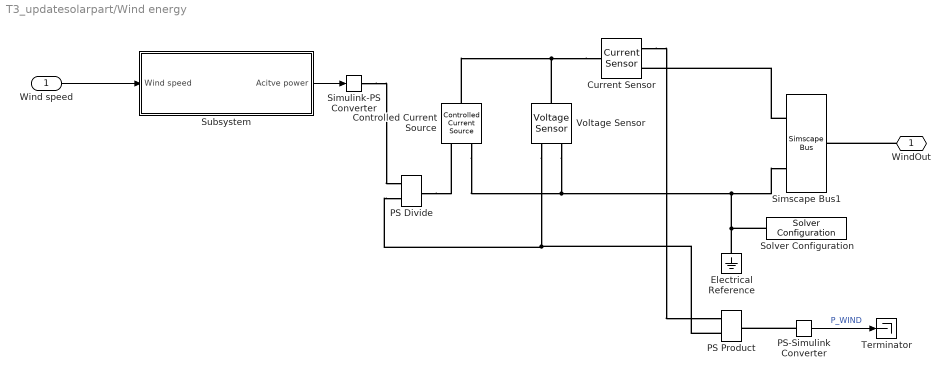
== system T3_updatesolarpart/Wind energy ==
  Wind speed : Inport
  Controlled Current Source : fl_lib/Electrical/Electrical Sources/Controlled Current Source
  Current Sensor : fl_lib/Electrical/Electrical Sensors/Current Sensor
  Electrical Reference : fl_lib/Electrical/Electrical Elements/Electrical Reference
  PS Divide : fl_lib/Physical Signals/Functions/PS Divide
  PS Product : fl_lib/Physical Signals/Functions/PS Product
  PS-Simulink Converter : nesl_utility/PS-Simulink Converter  PhysicalDomain=network_engine_domain  SubClassName=ps_output  LeftPortType=input  RightPortType=output  PseudoPeriodic=off  Frequencies=[]  VectorFormat=inherit  Unit=inherit  AffineConversion=off
  Simscape Bus1 : SimscapeBus  HierarchyStrings=High;Low
  Simulink-PS Converter : nesl_utility/Simulink-PS Converter  PhysicalDomain=network_engine_domain  SubClassName=ps_input  LeftPortType=input  RightPortType=output  PseudoPeriodic=off  Frequencies=[]  NoiseDistribution=none  NoiseParameters=[]  Unit=A*V  AffineConversion=off  FilteringAndDerivatives=provide  SimscapeFilterOrder=1  InputFilterTimeConstant=0.001  UdotUserProvided=0
  Solver Configuration : nesl_utility/Solver Configuration  PhysicalDomain=network_engine_domain  SubClassName=solver  LeftPortType=input  RightPortType=generic  Tones=[]  Harmonics=[]  SimulateNoise=off  Profile=off  UseLocalSampling=off  EnableSwitchedLinearOptims=on  FrequencyDomain=off  UseCCode=off  RelTol=0.001  AbsTol=0.001  MinStep=1e-09  ToWorkspace=off  RevertToSquareIcSolve=off  NumHomotopyIterations=100  PhasorMode=off  PhasorModeNumHarmonics=1  ConsistencySolver=NEWTON_XTOL_AFTER_FTOL  IndexReductionMethod=DerivativeReplacement  DoDC=off  ResidualTolerance=1e-09  ConsistencyTolSource=GLOBAL  ConsistencyAbsTol=0.001  ConsistencyRelTol=0.001  ConsistencyTolFactor=0.001  UseLocalSolver=off  LocalSolverChoice=NE_BACKWARD_EULER_ADVANCER  ResolveIndetEquations=on  FunctionEvalNumThread=1  LocalSolverSampleTime=0.001  DoFixedCost=off  MaxNonlinIter=3  MaxModeIter=2  ComputeImpulses=off  ImpulseIterations=2  LinearAlgebra=auto  LinearAlgebraNumThread=0  EquationFormulation=NE_TIME_EF  DelaysMemoryBudget=1024  AutomaticFiltering=on  FilteringTimeConstant=0.001  PartitionStorageMethod=AS_NEEDED  PartitionMemoryBudget=1024  PartitionMethod=ROBUST
  Subsystem : Subsystem
  Terminator : Terminator
  Voltage Sensor : fl_lib/Electrical/Electrical Sensors/Voltage Sensor
  WindOut : PMIOPort  Side=Right
  wires:
  PS-Simulink Converter/1 -> Terminator/1  "P_WIND"
  Subsystem/1(Acitve power) -> Simulink-PS Converter/1
  Wind speed/1 -> Subsystem/1(Wind speed)
  connections:
  PS Divide/RConn1 -- Controlled Current Source/RConn1
  Voltage Sensor/RConn2 -- Controlled Current Source/RConn2 -- Electrical Reference/LConn1 -- Solver Configuration/RConn1 -- Simscape Bus1/LConn2
  Simscape Bus1/LConn1 -- Current Sensor/RConn2
  PS Divide/LConn2 -- Voltage Sensor/RConn1 -- PS Product/LConn2
  PS-Simulink Converter/LConn1 -- PS Product/RConn1
  Current Sensor/LConn1 -- Controlled Current Source/LConn1 -- Voltage Sensor/LConn1
  Current Sensor/RConn1 -- PS Product/LConn1
  Simulink-PS Converter/RConn1 -- PS Divide/LConn1
  WindOut/RConn1 -- Simscape Bus1/RConn1

== system T3_updatesolarpart/Before t,off/Simscape2 ==
  Current Sensor : fl_lib/Electrical/Electrical Sensors/Current Sensor
  PS-S : nesl_utility/PS-Simulink Converter  PhysicalDomain=network_engine_domain  SubClassName=ps_output  LeftPortType=input  RightPortType=output  PseudoPeriodic=off  Frequencies=[]  VectorFormat=1-D array  Unit=A  AffineConversion=off
  + : PMIOPort  Side=Left
  - : PMIOPort  Port=2  Side=Left
  tag scope: ReplaceLine=global
  wires:
  PS-S/1 -> [ReplaceLine]  "current"
  connections:
  PS-S/LConn1 -- Current Sensor/RConn1
  Current Sensor/LConn1 -- +/RConn1
  -/RConn1 -- Current Sensor/RConn2

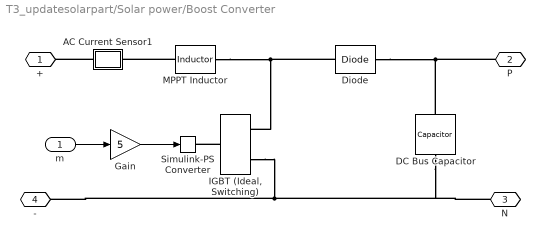
== system T3_updatesolarpart/Solar power/Boost Converter ==
  m : Inport
  AC Current Sensor1 : Subsystem
      mask Display: disp('i');
  DC Bus Capacitor : fl_lib/Electrical/Electrical Elements/Capacitor  c=1e-3 F  r=1e-6 Ohm  g=0 1/Ohm  i_specify=off  i_priority=None  i=0 A  i_nominal_specify=off  i_nominal_unit=A  i_nominal_value=1  v_specify=off  v_priority=None  v=0 V  v_nominal_specify=off  v_nominal_unit=V  v_nominal_value=1  vc_specify=on  vc_priority=High  vc=380 V  vc_nominal_specify=off  vc_nominal_unit=V  vc_nominal_value=1
  Diode : fl_lib/Electrical/Electrical Elements/Diode  Vf=0.6 V  Ron=0.3 Ohm  Goff=1e-8 1/Ohm  i_specify=off  i_priority=None  i=0 A  i_nominal_specify=off  i_nominal_unit=A  i_nominal_value=1  v_specify=off  v_priority=None  v=0 V  v_nominal_specify=off  v_nominal_unit=V  v_nominal_value=1
  Gain : Gain  Gain=5
  "IGBT (Ideal, Switching)" : ee_lib/Semiconductors & Converters/IGBT (Ideal, Switching)  port_option=ee.enum.controlport.ps  Vf=0.8 V  Ron=0.001 Ohm  Goff=1e-5 1/Ohm  Vth=2.5 V  diode_param=1  diode_Vf=0.8 V  diode_Ron=0.001 Ohm  diode_Goff=1e-5 1/Ohm  diode_C=50e-9 F  diode_iRM=-235 A  diode_iF=300 A  diode_idot=-50 A/us  diode_trr_param=1  diode_trr_factor=3  diode_trr=15 us  diode_Qrr=1500 s*uA  ice_specify=off  ice_priority=None  ice=0 A  ice_nominal_specify=off  ice_nominal_unit=A  ice_nominal_value=1  vce_specify=off  vce_priority=None  vce=0 V  vce_nominal_specify=off  vce_nominal_unit=V  vce_nominal_value=1  vge_specify=off  vge_priority=None  vge=0 V  vge_nominal_specify=off  vge_nominal_unit=V  vge_nominal_value=1  thermal_loss_option=ee.enum.converters.thermalLossOption.constantvalues  Von_data=[0, .1, .6, .8, 1, 1.3, 1.6, 2, 2.4; 0, .1, .7, 1, 1.2, 1.5, 1.9, 2.4, 2.8] V  Tj=[298.15, 398.15] K  Iout_data=[0, .1, 1, 5, 10, 20, 40, 70, 100] A  Eon_data=[0, .0024, .024, .12, .2, .48, 1.04, 2.16, 3.24; 0, .003, .03, .15, .25, .6, 1.3, 2.7, 4.05] * 1e-3 J  Eoff_data=[0, .0007, .0066, .033, .066, .17, .33, .83, 1.5; 0, .001, .01, .05, .1, .25, .5, 1.2, 2.2] * 1e-3 J  Tj_loss=[298.15, 398.15] K  Iout_data_loss=[0, .1, 1, 5, 10, 20, 40, 70, 100] A  Eon_scalar=22.86e-3 J  Eoff_scalar=17.14e-3 J  Voff=300 V  Iout_scalar=600 A  diodeModelType=ee.enum.converters.diodeModelType.pwl  diodeTableType=ee.enum.diode.tableType.IfMat  diode_IfMat=[.07, .12, .19, 1.75, 4.24, 7.32, 11.2; .16, .3, .72, 2.14, 4.02, 6.35, 9.12] A  diode_VfMat=[.9, 1.15, 1.25, 1.5, 1.75, 2.17, 2.6, 2.85; .58, .68, .75, 1.1, 1.38, 1.77, 2.27, 2.7] V  diode_TjVec=[25, 125] degC  diode_VfVec=[.5, .7, .9, 1.3, 1.7, 2.1, 2.5] V  diode_IfVec=[.1, .2, .5, 1, 2, 4, 7, 10] A  diode_Vr=-600 V  diode_Ls=150 nH  diode_Erec=0.03 J  thermal_network_parameterization=ee.enum.thermalNetworkTopology.external  Rth=[.08, .5] K/W  Rth_Cauer=[.08, .1, .5] K/W  Rth_Foster=[.08, .14, .22, .16] K/W  thermal_mass_parameterization=ee.enum.thermalNetwork.timeconstant  thermal_mass=[.01, .5] J/K  thermal_mass_Cauer=[.01, .1, .5] J/K  thermal_mass_Foster=[.001, .005, .05, .5] J/K  thermal_time_constant=[.001, .2] s  thermal_time_constant_Cauer=[.001, .1, .2] s  thermal_time_constant_Foster=[7e-05, .0007, .01, .08] s  thermal_mass_initial_temperatures=[25, 25] degC  thermal_mass_initial_temperatures_Cauer=[25, 25, 25] degC  junction_thermal_mass=0.01 J/K  Tvec_initial_Foster=[25, 25, 25, 25] degC  no_thermal_network=0  junction_temperature_specify=off  junction_temperature_priority=None  junction_temperature=25 degC  junction_temperature_nominal_specify=off  junction_temperature_nominal_unit=degC  junction_temperature_nominal_value=1  Qj_specify=off  Qj_priority=None  Qj=0 W  Qj_nominal_specify=off  Qj_nominal_unit=W  Qj_nominal_value=1
  MPPT Inductor : ee_lib/Passive/Inductor  l=0.0106 H  enable_L_tol=0  L_tol=5  tol_distribution=1  nSigma=4  r=0.1114 Ohm  g=1e-9 1/Ohm  enable_operating_limits=0  operating_limit_action=2  max_working_current=1 A  power_rating=1 W  enable_faults=0  fault_action=1  lambdaPercent=50  k_faulted=0.9999  turnsShort=0  openCct=0  groundShort=0  groundShortG=0 1/Ohm  tau_fault=1e-3 s  enable_temporal_fault=0  t_fault=1 s  enable_behavioral_fault=0  max_permissible_voltage=100 V  n_fail_on_voltage=1  max_permissible_current=1 A  t_fail_on_current=1 s  i_L_specify=on  i_L_priority=High  i_L=0 A  i_L_nominal_specify=off  i_L_nominal_unit=A  i_L_nominal_value=1
  Simulink-PS Converter : nesl_utility/Simulink-PS Converter  PhysicalDomain=network_engine_domain  SubClassName=ps_input  LeftPortType=input  RightPortType=output  PseudoPeriodic=off  Frequencies=[]  NoiseDistribution=none  NoiseParameters=[]  Unit=1  AffineConversion=off  FilteringAndDerivatives=provide  SimscapeFilterOrder=1  InputFilterTimeConstant=0.001  UdotUserProvided=0
  + : PMIOPort  Side=Left
  P : PMIOPort  Port=2  Side=Right
  N : PMIOPort  Port=3  Side=Right
  - : PMIOPort  Port=4  Side=Left
  wires:
  m/1 -> Gain/1
  Gain/1 -> Simulink-PS Converter/1
  connections:
  MPPT Inductor/LConn1 -- AC Current Sensor1/LConn1
  "IGBT (Ideal, Switching)"/RConn2 -- N/RConn1 -- DC Bus Capacitor/RConn1 -- -/RConn1
  AC Current Sensor1/RConn1 -- +/RConn1
  "IGBT (Ideal, Switching)"/LConn1 -- Simulink-PS Converter/RConn1
  MPPT Inductor/RConn1 -- "IGBT (Ideal, Switching)"/RConn1 -- Diode/LConn1
  DC Bus Capacitor/LConn1 -- Diode/RConn1 -- P/RConn1

== system T3_updatesolarpart/Solar power/I ==
  Current Sensor : fl_lib/Electrical/Electrical Sensors/Current Sensor
  PS-Simulink Converter : nesl_utility/PS-Simulink Converter  PhysicalDomain=network_engine_domain  SubClassName=ps_output  LeftPortType=input  RightPortType=output  PseudoPeriodic=off  Frequencies=[]  VectorFormat=inherit  Unit=inherit  AffineConversion=off
  + : PMIOPort  Side=Left
  - : PMIOPort  Port=2  Side=Right
  tag scope: Is=global
  wires:
  PS-Simulink Converter/1 -> [Is]
  connections:
  PS-Simulink Converter/LConn1 -- Current Sensor/RConn1
  Current Sensor/LConn1 -- +/RConn1
  Current Sensor/RConn2 -- -/RConn1

== system T3_updatesolarpart/Solar power/Subsystem ==
  note: Ns series panel
  Current-Controlled Current Source : fl_lib/Electrical/Electrical Sources/Current-Controlled Current Source  K=-1*(9-1)  i1_specify=off  i1_priority=None  i1=0 A  i1_nominal_specify=off  i1_nominal_unit=A  i1_nominal_value=1  i2_specify=off  i2_priority=None  i2=0 A  i2_nominal_specify=off  i2_nominal_unit=A  i2_nominal_value=1
      settings: InternalSimscapePortConfiguration="{\"Bottom\":[],\"Left\":[{\"id\":\"p1\",\"label\":\"+\",\"type\":\"foundation.electrical.electrical\"},{\"id\":\"head\",\"label\":\"\",\"type\":\"foundation.electrical.electrical\"}],\"Right\":[{\"id\":\"n1\",\"label\":\"-\",\"type\":\"foundation.electrical.electrical\"},{\"id\":\"tail\",\"label\":\"\",\"type\":\"foundation.electrical.electrical\"}],\"Top\":[]}"
  Current-Controlled Current Source- Scale panel current to Np parallel strings : fl_lib/Electrical/Electrical Sources/Current-Controlled Current Source  K=-1*(10-1)  i1_specify=off  i1_priority=None  i1=0 A  i1_nominal_specify=off  i1_nominal_unit=A  i1_nominal_value=1  i2_specify=off  i2_priority=None  i2=0 A  i2_nominal_specify=off  i2_nominal_unit=A  i2_nominal_value=1
      settings: InternalSimscapePortConfiguration="{\"Bottom\":[],\"Left\":[{\"id\":\"p1\",\"label\":\"+\",\"type\":\"foundation.electrical.electrical\"},{\"id\":\"head\",\"label\":\"\",\"type\":\"foundation.electrical.electrical\"}],\"Right\":[{\"id\":\"n1\",\"label\":\"-\",\"type\":\"foundation.electrical.electrical\"},{\"id\":\"tail\",\"label\":\"\",\"type\":\"foundation.electrical.electrical\"}],\"Top\":[]}"
  Solar Cell : ee_lib/Sources/Solar Cell  Tag={'toolbox/physmod/elec/library/m/ee_lib_parts';'Sources/Solar_Cell/Amerisolar/AS_6M30_HC_320W.xml'}  prm=1  Isc=10.00 A  Voc=0.673 V  Is=3.24823447983853e-07 A  Is2=9.37081970792037e-10 A  Iph=10.140005507508 A  Ir0=1000 W/m^2  ec=1.5  N2=2.60259908345858  Rs=0 Ohm  Rp=682.95993142779 Ohm  N_series=60  N_parallel=1  TIPH1=0.000499942933005141 1/K  EG=1.12 eV  TXIS1=4.23641510120988  TXIS2=16.2689137700667  TRS1=0.243341028305912  TRP1=0 % Parameter not set  Tmeas=25 degC  TFIXED=25 degC  thermal_mass=100 % Parameter not set J/K  initial_temperature=25 degC
      settings: AttributesFormatString=Amerisolar:AS_6M30_HC_320W
  Voltage-Controlled Voltage Source - Scale panel voltage to Ns series panel : fl_lib/Electrical/Electrical Sources/Voltage-Controlled Voltage Source  K=-1*(5-1)  v1_specify=off  v1_priority=None  v1=0 V  v1_nominal_specify=off  v1_nominal_unit=V  v1_nominal_value=1  v2_specify=off  v2_priority=None  v2=0 V  v2_nominal_specify=off  v2_nominal_unit=V  v2_nominal_value=1
      settings: InternalSimscapePortConfiguration="{\"Bottom\":[],\"Left\":[{\"id\":\"p1\",\"label\":\"+\",\"type\":\"foundation.electrical.electrical\"},{\"id\":\"p2\",\"label\":\"+\",\"type\":\"foundation.electrical.electrical\"}],\"Right\":[{\"id\":\"n1\",\"label\":\"-\",\"type\":\"foundation.electrical.electrical\"},{\"id\":\"n2\",\"label\":\"-\",\"type\":\"foundation.electrical.electrical\"}],\"Top\":[]}"
  Iradiance : PMIOPort  Side=Left
  + : PMIOPort  Port=2  Side=Right
  - : PMIOPort  Port=3  Side=Right
  connections:
  Solar Cell/LConn2 -- Current-Controlled Current Source/LConn1
  Voltage-Controlled Voltage Source - Scale panel voltage to Ns series panel/RConn1 -- Current-Controlled Current Source/RConn1 -- Current-Controlled Current Source/RConn2 -- Voltage-Controlled Voltage Source - Scale panel voltage to Ns series panel/RConn2
  Iradiance/RConn1 -- Solar Cell/LConn1
  Current-Controlled Current Source- Scale panel current to Np parallel strings/LConn2 -- -/RConn1 -- Solar Cell/RConn1 -- Current-Controlled Current Source/LConn2 -- Voltage-Controlled Voltage Source - Scale panel voltage to Ns series panel/LConn1
  Current-Controlled Current Source- Scale panel current to Np parallel strings/RConn2 -- +/RConn1 -- Current-Controlled Current Source- Scale panel current to Np parallel strings/RConn1
  Current-Controlled Current Source- Scale panel current to Np parallel strings/LConn1 -- Voltage-Controlled Voltage Source - Scale panel voltage to Ns series panel/LConn2

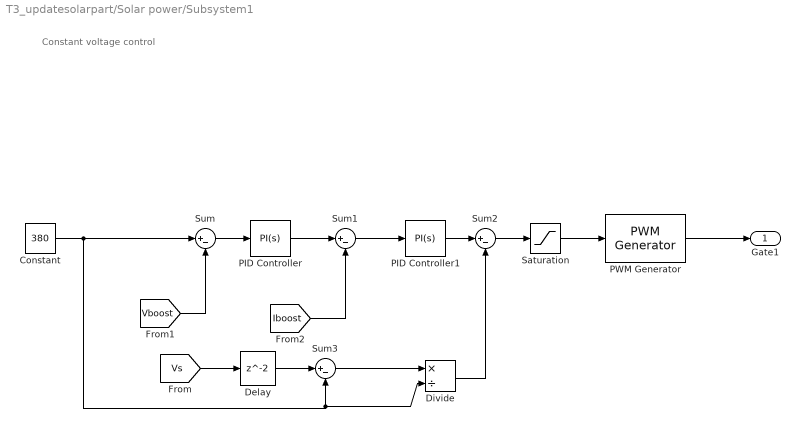
== system T3_updatesolarpart/Solar power/Subsystem1 ==
  note: Constant voltage control
  Constant : Constant  Value=380
  Delay : Delay
  Divide : Product  Inputs=*/
  PID Controller : slpidlib/PID Controller  Controller=PI  Form=Parallel  TimeDomain=Continuous-time  UseExternalTs=off  SampleTime=-1  IntegratorMethod=Forward Euler  FilterMethod=Forward Euler  ControllerParametersSource=internal  P=300  I=0.001  UseKiTs=off  D=0  N=100  UseFilter=on  TunerSelectOption=Transfer Function Based (PID Tuner App)  InitialConditionSource=internal  InitialConditionForIntegrator=0  InitialConditionForFilter=0  DifferentiatorICPrevScaledInput=0  ExternalReset=none  TrackingMode=off  Kt=1  LimitOutput=on  SatLimitsSource=internal  UpperSaturationLimit=11  LowerSaturationLimit=0  LinearizeAsGain=on  AntiWindupMode=none  Kb=1  LimitIntegrator=off  UpperIntegratorSaturationLimit=inf  LowerIntegratorSaturationLimit=-inf  POutMin=[]  POutMax=[]  IOutMin=[]  IOutMax=[]  DOutMin=[]  DOutMax=[]  NOutMin=[]  NOutMax=[]  SumOutMin=[]  SumOutMax=[]  SaturationOutMin=[]  SaturationOutMax=[]  PParamMin=[]  PParamMax=[]  IParamMin=[]  IParamMax=[]  DParamMin=[]  DParamMax=[]  NParamMin=[]  NParamMax=[]  KbParamMin=[]  KbParamMax=[]  KtParamMin=[]  KtParamMax=[]  KbOutMin=[]  KbOutMax=[]  KtOutMin=[]  KtOutMax=[]  IntegratorOutMin=[]  IntegratorOutMax=[]  FilterOutMin=[]  FilterOutMax=[]  SumI1OutMin=[]  SumI1OutMax=[]  SumI2OutMin=[]  SumI2OutMax=[]  SumI3OutMin=[]  SumI3OutMax=[]  SumI4OutMin=[]  SumI4OutMax=[]  SumDOutMin=[]  SumDOutMax=[]  DifferentiatorOutMin=[]  DifferentiatorOutMax=[]  FilterDiffOutCoefMin=[]  FilterDiffOutCoefMax=[]  ReciprocalOutMin=[]  ReciprocalOutMax=[]  SumDenOutMin=[]  SumDenOutMax=[]  SumNumOutMin=[]  SumNumOutMax=[]  DivideOutMin=[]  DivideOutMax=[]  UdiffTsProdOutMin=[]  UdiffTsProdOutMax=[]  NTsProdOutMin=[]  NTsProdOutMax=[]  UintegralTsProdOutMin=[]  UintegralTsProdOutMax=[]  UngainTsProdOutMin=[]  UngainTsProdOutMax=[]  ClampingZeroOutDataTypeStr=Inherit: Inherit via back propagation  ClampingZeroOutMin=[]  ClampingZeroOutMax=[]  FilterDenConstantOutDataTypeStr=Inherit: Inherit via back propagation  FilterDenConstantOutMin=[]  FilterDenConstantOutMax=[]  PCopyOutDataTypeStr=Inherit: Inherit via back propagation  PCopyOutMin=[]  PCopyOutMax=[]  NCopyOutDataTypeStr=Inherit: Inherit via back propagation  NCopyOutMin=[]  NCopyOutMax=[]  IntegratorContinuousStateAttributes=''  IntegratorStateMustResolveToSignalObject=off  IntegratorRTWStateStorageClass=Auto  FilterContinuousStateAttributes=''  FilterStateMustResolveToSignalObject=off  FilterRTWStateStorageClass=Auto  ParallelPVariant=InternalParameters  IdealPVariant=Disabled  IVariant=InternalParameters  DVariant=Disabled  IntegratorVariant=Continuous  SatVariant=Enabled  AWVariant=Passthrough  PCopyVariant=Disabled  TRVariant=Disabled  FdbkBlocksVariant=Forward  IdealPFdbkVariant=Disabled  SatFdbkVariant=Disabled  DerivativeFilterVariant=Disabled  NVariant=Disabled  NCopyVariant=Disabled_SignalSpec  FilterICVariant=Disabled  IntegratorICVariant=InternalICs  ExternalResetVariant=Disabled  TRSumVariant=Passthrough  SumFdbkVariant=Disabled  SumVariant=Sum_PI  TsampFilterVariant=InternalTs  TsampNgainVariant=Passthrough  TsampIntegralVariant=Passthrough  ExternalSaturationOutDataTypeStr=Inherit: Same as second input
  PID Controller1 : slpidlib/PID Controller  Controller=PI  Form=Parallel  TimeDomain=Continuous-time  UseExternalTs=off  SampleTime=-1  IntegratorMethod=Forward Euler  FilterMethod=Forward Euler  ControllerParametersSource=internal  P=0.5  I=1  UseKiTs=off  D=0  N=100  UseFilter=on  TunerSelectOption=Transfer Function Based (PID Tuner App)  InitialConditionSource=internal  InitialConditionForIntegrator=0  InitialConditionForFilter=0  DifferentiatorICPrevScaledInput=0  ExternalReset=none  TrackingMode=off  Kt=1  LimitOutput=off  SatLimitsSource=internal  UpperSaturationLimit=inf  LowerSaturationLimit=-inf  LinearizeAsGain=on  AntiWindupMode=none  Kb=1  LimitIntegrator=off  UpperIntegratorSaturationLimit=inf  LowerIntegratorSaturationLimit=-inf  POutMin=[]  POutMax=[]  IOutMin=[]  IOutMax=[]  DOutMin=[]  DOutMax=[]  NOutMin=[]  NOutMax=[]  SumOutMin=[]  SumOutMax=[]  SaturationOutMin=[]  SaturationOutMax=[]  PParamMin=[]  PParamMax=[]  IParamMin=[]  IParamMax=[]  DParamMin=[]  DParamMax=[]  NParamMin=[]  NParamMax=[]  KbParamMin=[]  KbParamMax=[]  KtParamMin=[]  KtParamMax=[]  KbOutMin=[]  KbOutMax=[]  KtOutMin=[]  KtOutMax=[]  IntegratorOutMin=[]  IntegratorOutMax=[]  FilterOutMin=[]  FilterOutMax=[]  SumI1OutMin=[]  SumI1OutMax=[]  SumI2OutMin=[]  SumI2OutMax=[]  SumI3OutMin=[]  SumI3OutMax=[]  SumI4OutMin=[]  SumI4OutMax=[]  SumDOutMin=[]  SumDOutMax=[]  DifferentiatorOutMin=[]  DifferentiatorOutMax=[]  FilterDiffOutCoefMin=[]  FilterDiffOutCoefMax=[]  ReciprocalOutMin=[]  ReciprocalOutMax=[]  SumDenOutMin=[]  SumDenOutMax=[]  SumNumOutMin=[]  SumNumOutMax=[]  DivideOutMin=[]  DivideOutMax=[]  UdiffTsProdOutMin=[]  UdiffTsProdOutMax=[]  NTsProdOutMin=[]  NTsProdOutMax=[]  UintegralTsProdOutMin=[]  UintegralTsProdOutMax=[]  UngainTsProdOutMin=[]  UngainTsProdOutMax=[]  ClampingZeroOutDataTypeStr=Inherit: Inherit via back propagation  ClampingZeroOutMin=[]  ClampingZeroOutMax=[]  FilterDenConstantOutDataTypeStr=Inherit: Inherit via back propagation  FilterDenConstantOutMin=[]  FilterDenConstantOutMax=[]  PCopyOutDataTypeStr=Inherit: Inherit via back propagation  PCopyOutMin=[]  PCopyOutMax=[]  NCopyOutDataTypeStr=Inherit: Inherit via back propagation  NCopyOutMin=[]  NCopyOutMax=[]  IntegratorContinuousStateAttributes=''  IntegratorStateMustResolveToSignalObject=off  IntegratorRTWStateStorageClass=Auto  FilterContinuousStateAttributes=''  FilterStateMustResolveToSignalObject=off  FilterRTWStateStorageClass=Auto  ParallelPVariant=InternalParameters  IdealPVariant=Disabled  IVariant=InternalParameters  DVariant=Disabled  IntegratorVariant=Continuous  SatVariant=Disabled  AWVariant=Passthrough  PCopyVariant=Disabled  TRVariant=Disabled  FdbkBlocksVariant=Forward  IdealPFdbkVariant=Disabled  SatFdbkVariant=Disabled  DerivativeFilterVariant=Disabled  NVariant=Disabled  NCopyVariant=Disabled_SignalSpec  FilterICVariant=Disabled  IntegratorICVariant=InternalICs  ExternalResetVariant=Disabled  TRSumVariant=Passthrough  SumFdbkVariant=Disabled  SumVariant=Sum_PI  TsampFilterVariant=InternalTs  TsampNgainVariant=Passthrough  TsampIntegralVariant=Passthrough  ExternalSaturationOutDataTypeStr=Inherit: Same as second input
  PWM Generator : eePwmGenerator/PWM Generator  CarrCount=Up  Tper=1/20e3  Tdelay=0  Ts=1/(10*20e3)
  Saturation : Saturate  UpperLimit=1  LowerLimit=0
  Sum{,1..3} (4 alike) : Sum  Inputs=|+-
  Gate1 : Outport
  wires:
  Sum1/1 -> PID Controller1/1
  PID Controller1/1 -> Sum2/1
  PID Controller/1 -> Sum1/1
  [Vs] -> Delay/1
  Sum2/1 -> Saturation/1
  [Iboost] -> Sum1/2
  Sum/1 -> PID Controller/1
  [Vboost] -> Sum/2
  Saturation/1 -> PWM Generator/1
  PWM Generator/1 -> Gate1/1
  Sum3/1 -> Divide/1
  Constant/1 -> Sum3/2, Divide/2, Sum/1
  Divide/1 -> Sum2/2
  Delay/1 -> Sum3/1

== system T3_updatesolarpart/Solar power/Subsystem2 ==
  PS-Simulink Converter : nesl_utility/PS-Simulink Converter  PhysicalDomain=network_engine_domain  SubClassName=ps_output  LeftPortType=input  RightPortType=output  PseudoPeriodic=off  Frequencies=[]  VectorFormat=inherit  Unit=inherit  AffineConversion=off
  Voltage Sensor : fl_lib/Electrical/Electrical Sensors/Voltage Sensor
  - : PMIOPort  Side=Right
  + : PMIOPort  Port=2  Side=Left
  tag scope: Vboost=global
  wires:
  PS-Simulink Converter/1 -> [Vboost]
  connections:
  PS-Simulink Converter/LConn1 -- Voltage Sensor/RConn1
  Voltage Sensor/LConn1 -- +/RConn1
  Voltage Sensor/RConn2 -- -/RConn1
